simulink model "ddr4_isov"  (R2025a)
settings: Solver=VariableStepAuto  StartTime=0.0  StopTime=10.0  RelTol=1e-3
libraries: hdlBasic x10
settings Model: Creator=qwerty40  LastModifiedBy=mcb
settings SolverCC: AlgebraicLoopSolver=TrustRegion
settings DataIOCC: ReturnWorkspaceOutputs=off
settings DebuggingCC: UnconnectedInputMsg=warning  UnconnectedOutputMsg=warning  UnconnectedLineMsg=warning  ArithmeticOperatorsInVariantConditions=warning
settings ModelReferenceCC: EnableRefExpFcnMdlSchedulingChecks=on
settings SFSimCC: SimUseLocalCustomCode=off  CustomCodeUndefinedFunction=UseInterfaceOnly
settings RTWCC: RTWUseLocalCustomCode=off  GPUComputeCapability=3.5  DLArmComputeVersion=19.05
settings CodeAppCC: StateflowObjectComments=on

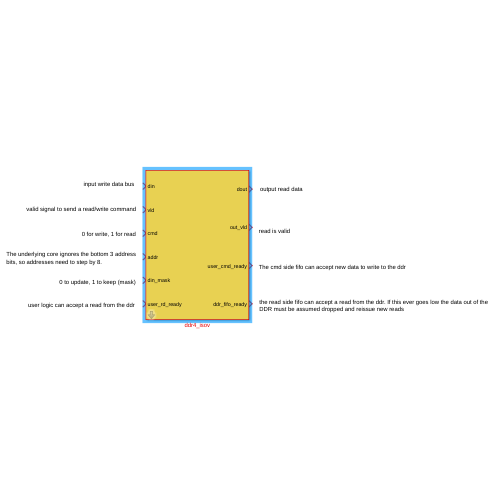
[thumbnail: Simulink's stored preview of the top-level diagram]
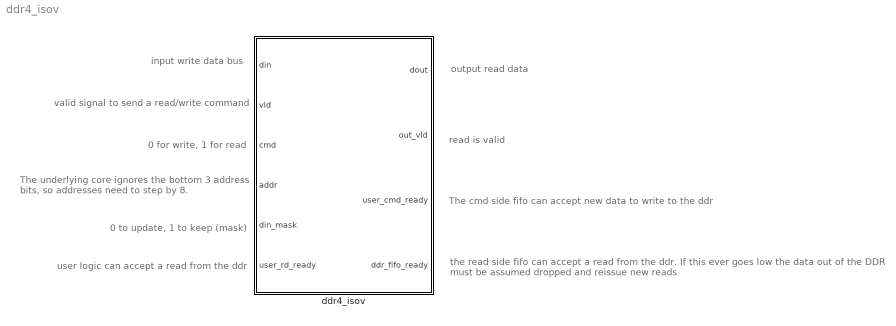
== system ddr4_isov ==
  note: output read data
  note: read is valid
  note: valid signal to send a read/write command
  note: input write data bus
  note: The cmd side fifo can accept new data to write to the ddr
  note: the read side fifo can accept a read from the ddr. If this ever goes low the data out of the DDR must be assumed dropped and reissue new reads
  note: user logic can accept a read from the ddr
  note: 0 to update, 1 to keep (mask)
  note: 0 for write, 1 for read
  note: The underlying core ignores the bottom 3 address
      | bits, so addresses need to step by 8.
  ddr4_isov : Subsystem  Tag=xps:ddr4_isov  mask(ddr4){width=512, sample_period=1}
      mask prompts: width "DDR Bitwidth"; sample_period "Sample Period"
      mask init:
      | ddr4_isov_mask(gcb);
      mask TypeOptions width: 512

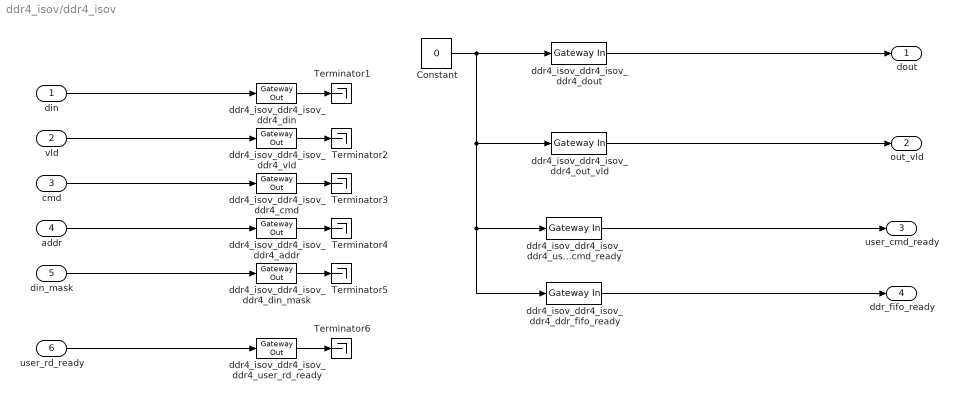
== system ddr4_isov/ddr4_isov ==
  din : Inport
  vld : Inport  Port=2
  cmd : Inport  Port=3
  addr : Inport  Port=4
  din_mask : Inport  Port=5
  user_rd_ready : Inport  Port=6
  Constant : Constant  Value=0
  Terminator{1..6} (6 alike) : Terminator
  ddr4_isov_ddr4_isov_ddr4_addr : hdlBasic/Gateway Out  inherit_from_input=off  bool_to_boolean=off  hdl_port=on  rows=1  columns=1  UseAsDAC=off  DACChannel='1'  interface=None  automatic_assignment=on  address_offset=hex2dec('00')  intf_name=''  intf_description=''  timing_constraint=None  locs_specified=off  LOCs={}  io_standard={}  XmcBlockStatus=1  maskContainerNames=group4  block_type=gatewayout  block_config=sysgen:gateway_out_config  block_width_w=590  block_height_w=620  block_width=620  block_height=750
  ddr4_isov_ddr4_isov_ddr4_cmd : hdlBasic/Gateway Out  inherit_from_input=off  bool_to_boolean=off  hdl_port=on  rows=1  columns=1  UseAsDAC=off  DACChannel='1'  interface=None  automatic_assignment=on  address_offset=hex2dec('00')  intf_name=''  intf_description=''  timing_constraint=None  locs_specified=off  LOCs={}  io_standard={}  XmcBlockStatus=1  maskContainerNames=group4  block_type=gatewayout  block_config=sysgen:gateway_out_config  block_width_w=590  block_height_w=620  block_width=620  block_height=750
  ddr4_isov_ddr4_isov_ddr4_ddr_fifo_ready : hdlBasic/Gateway In  gui_display_data_type=Boolean  arith_type=Boolean  n_bits=8*32  bin_pt=0  preci_type=Single  exp_width=8  frac_width=24  rows=1  columns=1  quantization=Truncate  overflow=Wrap  period=sample_period  UseAsADC=off  ADCChannel='1'  interface=None  automatic_assignment=on  address_offset=hex2dec('00')  intf_name=''  intf_description=''  default_value=0  timing_constraint=None  locs_specified=off  LOCs={}  io_standard={}  inherit_from_input=off  hdl_port=on  XmcBlockStatus=1  maskContainerNames=group4  block_type=gatewayin  block_config=sysgen:gateway_in_config  block_width_w=590  block_height_w=620  block_width=640  block_height=850
  ddr4_isov_ddr4_isov_ddr4_din : hdlBasic/Gateway Out  inherit_from_input=off  bool_to_boolean=off  hdl_port=on  rows=1  columns=1  UseAsDAC=off  DACChannel='1'  interface=None  automatic_assignment=on  address_offset=hex2dec('00')  intf_name=''  intf_description=''  timing_constraint=None  locs_specified=off  LOCs={}  io_standard={}  XmcBlockStatus=1  maskContainerNames=group4  block_type=gatewayout  block_config=sysgen:gateway_out_config  block_width_w=590  block_height_w=620  block_width=620  block_height=750
  ddr4_isov_ddr4_isov_ddr4_din_mask : hdlBasic/Gateway Out  inherit_from_input=off  bool_to_boolean=off  hdl_port=on  rows=1  columns=1  UseAsDAC=off  DACChannel='1'  interface=None  automatic_assignment=on  address_offset=hex2dec('00')  intf_name=''  intf_description=''  timing_constraint=None  locs_specified=off  LOCs={}  io_standard={}  XmcBlockStatus=1  maskContainerNames=group4  block_type=gatewayout  block_config=sysgen:gateway_out_config  block_width_w=590  block_height_w=620  block_width=620  block_height=750
  ddr4_isov_ddr4_isov_ddr4_dout : hdlBasic/Gateway In  gui_display_data_type=Fixed-point  arith_type=Unsigned  n_bits=8*64  bin_pt=0  preci_type=Single  exp_width=8  frac_width=24  rows=1  columns=1  quantization=Truncate  overflow=Wrap  period=sample_period  UseAsADC=off  ADCChannel='1'  interface=None  automatic_assignment=on  address_offset=hex2dec('00')  intf_name=''  intf_description=''  default_value=0  timing_constraint=None  locs_specified=off  LOCs={}  io_standard={}  inherit_from_input=off  hdl_port=on  XmcBlockStatus=1  maskContainerNames=group4  block_type=gatewayin  block_config=sysgen:gateway_in_config  block_width_w=590  block_height_w=620  block_width=640  block_height=850
  ddr4_isov_ddr4_isov_ddr4_out_vld : hdlBasic/Gateway In  gui_display_data_type=Boolean  arith_type=Boolean  n_bits=144  bin_pt=0  preci_type=Single  exp_width=8  frac_width=24  rows=1  columns=1  quantization=Truncate  overflow=Wrap  period=sample_period  UseAsADC=off  ADCChannel='1'  interface=None  automatic_assignment=on  address_offset=hex2dec('00')  intf_name=''  intf_description=''  default_value=0  timing_constraint=None  locs_specified=off  LOCs={}  io_standard={}  inherit_from_input=off  hdl_port=on  XmcBlockStatus=1  maskContainerNames=group4  block_type=gatewayin  block_config=sysgen:gateway_in_config  block_width_w=590  block_height_w=620  block_width=640  block_height=850
  ddr4_isov_ddr4_isov_ddr4_user_cmd_ready : hdlBasic/Gateway In  gui_display_data_type=Boolean  arith_type=Boolean  n_bits=8*32  bin_pt=0  preci_type=Single  exp_width=8  frac_width=24  rows=1  columns=1  quantization=Truncate  overflow=Wrap  period=sample_period  UseAsADC=off  ADCChannel='1'  interface=None  automatic_assignment=on  address_offset=hex2dec('00')  intf_name=''  intf_description=''  default_value=0  timing_constraint=None  locs_specified=off  LOCs={}  io_standard={}  inherit_from_input=off  hdl_port=on  XmcBlockStatus=1  maskContainerNames=group4  block_type=gatewayin  block_config=sysgen:gateway_in_config  block_width_w=590  block_height_w=620  block_width=640  block_height=850
  ddr4_isov_ddr4_isov_ddr4_user_rd_ready : hdlBasic/Gateway Out  inherit_from_input=off  bool_to_boolean=off  hdl_port=on  rows=1  columns=1  UseAsDAC=off  DACChannel='1'  interface=None  automatic_assignment=on  address_offset=hex2dec('00')  intf_name=''  intf_description=''  timing_constraint=None  locs_specified=off  LOCs={}  io_standard={}  XmcBlockStatus=1  maskContainerNames=group4  block_type=gatewayout  block_config=sysgen:gateway_out_config  block_width_w=590  block_height_w=620  block_width=620  block_height=750
  ddr4_isov_ddr4_isov_ddr4_vld : hdlBasic/Gateway Out  inherit_from_input=off  bool_to_boolean=off  hdl_port=on  rows=1  columns=1  UseAsDAC=off  DACChannel='1'  interface=None  automatic_assignment=on  address_offset=hex2dec('00')  intf_name=''  intf_description=''  timing_constraint=None  locs_specified=off  LOCs={}  io_standard={}  XmcBlockStatus=1  maskContainerNames=group4  block_type=gatewayout  block_config=sysgen:gateway_out_config  block_width_w=590  block_height_w=620  block_width=620  block_height=750
  dout : Outport
  out_vld : Outport  Port=2
  user_cmd_ready : Outport  Port=3
  ddr_fifo_ready : Outport  Port=4
  wires:
  din_mask/1 -> ddr4_isov_ddr4_isov_ddr4_din_mask/1
  addr/1 -> ddr4_isov_ddr4_isov_ddr4_addr/1
  cmd/1 -> ddr4_isov_ddr4_isov_ddr4_cmd/1
  din/1 -> ddr4_isov_ddr4_isov_ddr4_din/1
  ddr4_isov_ddr4_isov_ddr4_out_vld/1 -> out_vld/1
  vld/1 -> ddr4_isov_ddr4_isov_ddr4_vld/1
  ddr4_isov_ddr4_isov_ddr4_din/1 -> Terminator1/1
  ddr4_isov_ddr4_isov_ddr4_vld/1 -> Terminator2/1
  ddr4_isov_ddr4_isov_ddr4_cmd/1 -> Terminator3/1
  ddr4_isov_ddr4_isov_ddr4_addr/1 -> Terminator4/1
  ddr4_isov_ddr4_isov_ddr4_din_mask/1 -> Terminator5/1
  Constant/1 -> ddr4_isov_ddr4_isov_ddr4_dout/1, ddr4_isov_ddr4_isov_ddr4_ddr_fifo_ready/1, ddr4_isov_ddr4_isov_ddr4_user_cmd_ready/1, ddr4_isov_ddr4_isov_ddr4_out_vld/1
  ddr4_isov_ddr4_isov_ddr4_dout/1 -> dout/1
  ddr4_isov_ddr4_isov_ddr4_user_cmd_ready/1 -> user_cmd_ready/1
  user_rd_ready/1 -> ddr4_isov_ddr4_isov_ddr4_user_rd_ready/1
  ddr4_isov_ddr4_isov_ddr4_user_rd_ready/1 -> Terminator6/1
  ddr4_isov_ddr4_isov_ddr4_ddr_fifo_ready/1 -> ddr_fifo_ready/1
